simulink model "H_Bridge"  (R2024a)
settings: Solver=VariableStepAuto  StartTime=0.0  StopTime=0.2  RelTol=1e-3
libraries: spsDCVoltageSourceLib x1, spsFullBridgeMMCExternalDCLinksLib x1, eePwmGeneratorMultilevel x1, spsSeriesRLCBranchLib x1, spsVoltageMeasurementLib x1, sps_lib x1
settings Model: Creator=MEET  LastModifiedBy=MEET

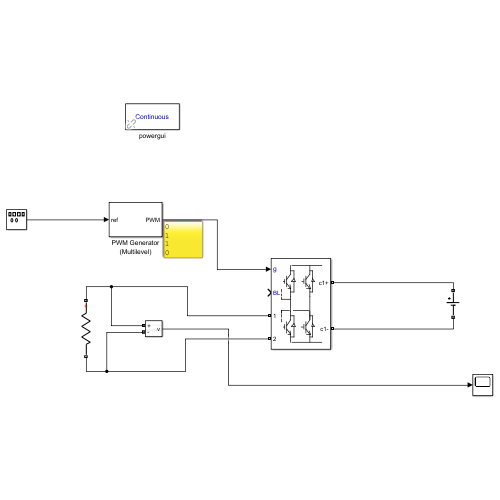
[thumbnail: Simulink's stored preview of the top-level diagram]
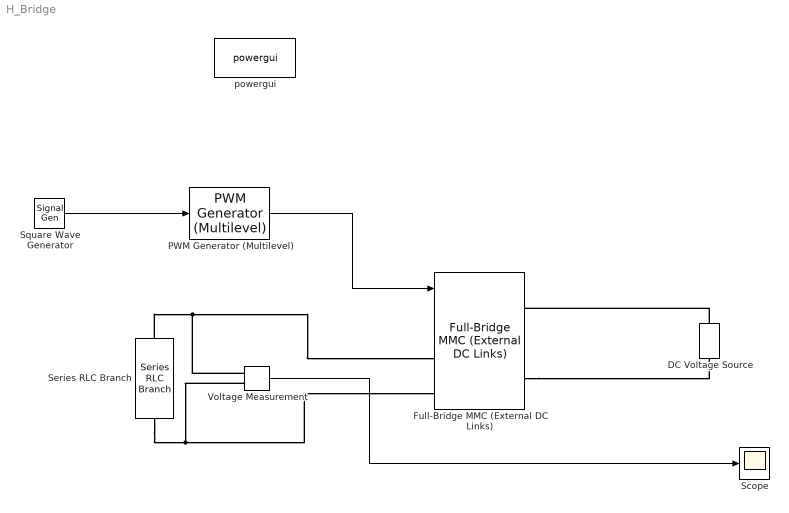
== system H_Bridge ==
  DC Voltage Source : spsDCVoltageSourceLib/DC Voltage Source  Amplitude=100  Measurements=None
  Full-Bridge MMC (External DC Links) : spsFullBridgeMMCExternalDCLinksLib/Full-Bridge MMC (External DC Links)  ModelType=Switching devices  n=1  Ron=1e-3  Rs=1e6  Cs=inf  Ron_Diode=1e-3  Rs_Diode=1e6  Cs_Diode=inf  Vf_Diode=1e-3  Rs_CurrentSource=inf  Ts=10e-6
      settings: LibrarySourceBlock=|
      | sps_lib/Power Electronics/Full-Bridge MMC
      | (External DC Links)
  PWM Generator (Multilevel) : eePwmGeneratorMultilevel/PWM Generator (Multilevel)  topology=Full-bridge  Nsm=1  Tper=0.001  Ts=5e-5
      settings: LibrarySourceBlock=|
      | ee_sl_lib/Pulse Width
      | Modulation/PWM Generator
      | (Multilevel)
  Scope : Scope
  Series RLC Branch : spsSeriesRLCBranchLib/Series RLC Branch  LConnTagsString=__new0  RConnTagsString=__new0  BranchType=R  Resistance=1  Inductance=1e-3  SetiL0=off  InitialCurrent=0  Capacitance=1e-6  Setx0=off  InitialVoltage=0  Measurements=None
  Square Wave Generator : SignalGenerator  WaveForm=square  Frequency=100*pi  Units=rad/sec
  Voltage Measurement : spsVoltageMeasurementLib/Voltage Measurement  PhasorSimulation=off  OutputType=Complex  PSBequivalent=0
  powergui : sps_lib/powergui  Priority=1  SimulationMode=Continuous  SampleTime=50e-6  frequency=60  Iterations=50  frequencyindice=0  Pbase=100e6  ErrMax=1e-4  UnitsV=kV  UnitsW=MW  buscounter=0  FunctionMessages=off  echomessages=off  EnableUseOfTLC=off  CurrentSourceSwitches=off  DisableSnubberDevices=off  DisableRonSwitches=off  DisableVfSwitches=off  DisplayEquations=off  AutomaticDiscreteSolvers=off  SolverType=Tustin/Backward Euler (TBE)  Interpol=off  ExternalGateDelay=off  methode=off  Ts=100  x0status=blocks  SPID=on  SwTol=0  HookPort=off  NonlinearTolerance=1e-4  nMaxIteration=100  ContinueOnMaxIteration=off  RestoreLinks=warning  ResistiveCurrentMeasurement=off  Frange=[0:2:500]  Ylog=off  Xlog=on  ShowGrid=off  save=off  variable=ZData  structure=0  ZoomFFT=off  StartTime=0.0  cycles=1  DisplayStyle=1  fundamental=60  FreqAxis=off  MaxFrequency=1000  frequencyindicesteady=1  RmsSteady=1  display=off
  wires:
  PWM Generator (Multilevel)/1 -> Full-Bridge MMC (External DC Links)/1
  Square Wave Generator/1 -> PWM Generator (Multilevel)/1
  Voltage Measurement/1 -> Scope/1
  connections:
  DC Voltage Source/RConn1 -- Full-Bridge MMC (External DC Links)/RConn1
  Full-Bridge MMC (External DC Links)/RConn2 -- DC Voltage Source/LConn1
  Series RLC Branch/LConn1 -- Voltage Measurement/LConn1 -- Full-Bridge MMC (External DC Links)/LConn1
  Series RLC Branch/RConn1 -- Voltage Measurement/LConn2 -- Full-Bridge MMC (External DC Links)/LConn2
